simulink model "questao3"  (R2023a)
settings: Solver=VariableStepAuto  StartTime=0.0  StopTime=100  RelTol=1e-3
values from neighbouring files (symbols this model uses):
  B = 0.1    [Trab1_real.m]    (also in questao5.m)
  i0 = 0    [Trab1_real.m]    (also in questao5.m)
  J = 1    [Trab1_real.m]    (also in questao5.m)
  K = 1/3    (= 0.333333333333)    [Trab1_real.m]    (also in questao5.m)
  L = 0.5    [Trab1_real.m]    (also in questao5.m)
  R = 10    [Trab1_real.m]    (also in questao5.m)
settings Model: Creator=pedro  LastModifiedBy=pedro

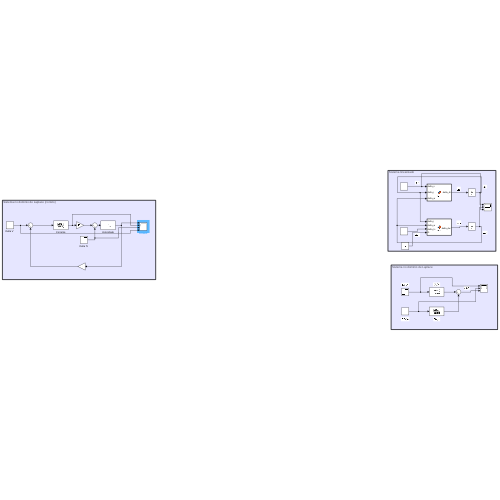
[thumbnail: Simulink's stored preview of the top-level diagram]
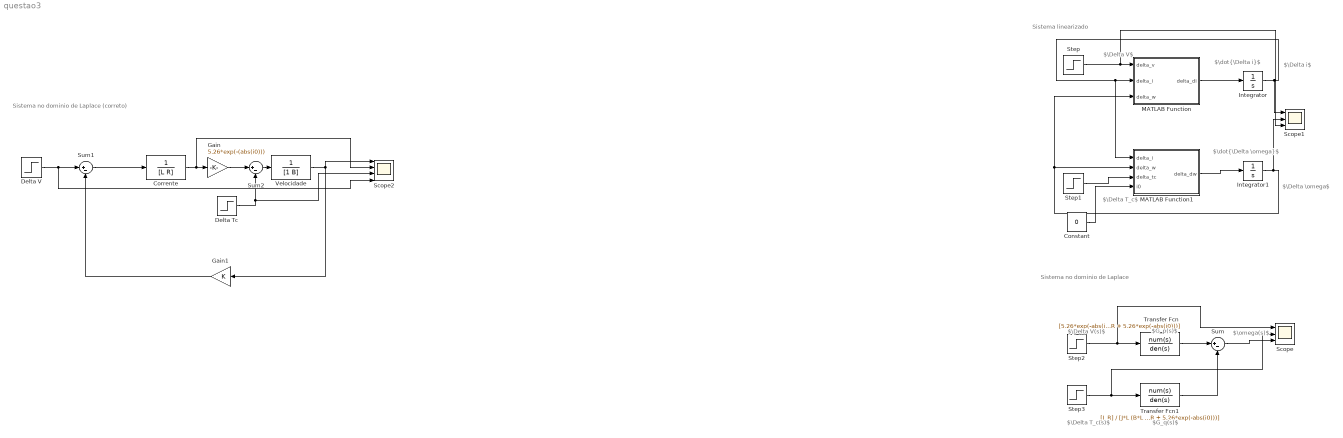
== system questao3 ==
  note: Sistema no dominio de Laplace (correto)
  note: Sistema no dominio de Laplace
  note: $\omega(s)$
  note: $G_q(s)$
  note: $G_p(s)$
  note: $\Delta T_c(s)$
  note: $\Delta V(s)$
  note: $\Delta T_c$
  note: $\Delta V$
  note: $\Delta \omega$
  note: $\dot{\Delta \omega}$
  note: $\Delta i$
  note: $\dot{\Delta i}$
  note: Sistema linearizado
  Constant : Constant  Value=0
  Corrente : TransferFcn  Denominator=[L R]
  Delta Tc : Step  Time=10  After=0.25  SampleTime=0
  "Delta V " : Step  Time=10  After=2  SampleTime=0
  Gain : Gain  Gain=5.26*exp(-(abs(i0)))
  Gain1 : Gain  Gain=K
  Integrator : Integrator
  Integrator1 : Integrator
  MATLAB Function : MATLAB Function  TreatAsAtomicUnit=on
  MATLAB Function1 : MATLAB Function  TreatAsAtomicUnit=on
  Scope : Scope  NumInputPorts=3
  Scope1 : Scope  NumInputPorts=3
  Scope2 : Scope  NumInputPorts=4
  Step : Step  Time=10  After=2  SampleTime=0
  Step1 : Step  Time=10  After=0.25  SampleTime=0
  Step2 : Step  Time=10  After=2  SampleTime=0
  Step3 : Step  Time=10  After=0.25  SampleTime=0
  Sum : Sum  Inputs=|+-
  Sum1 : Sum  Inputs=|+-
  Sum2 : Sum  Inputs=|+-
  Transfer Fcn : TransferFcn  Numerator=[5.26*exp(-abs(i0))]  Denominator=[J*L (B*L + R*J) (B*R + 5.26*exp(-abs(i0)))]
  Transfer Fcn1 : TransferFcn  Numerator=[L R]  Denominator=[J*L (B*L + R*J) (B*R + 5.26*exp(-abs(i0)))]
  Velocidade : TransferFcn  Denominator=[1 B]
  wires:
  MATLAB Function/1(delta_di) -> Integrator/1
  Step/1 -> Scope1/3, MATLAB Function/1(delta_v)
  Integrator/1 -> MATLAB Function1/1(delta_i), MATLAB Function/2(delta_i), Scope1/1
  Step1/1 -> MATLAB Function1/3(delta_tc)
  MATLAB Function1/1(delta_dw) -> Integrator1/1
  Integrator1/1 -> Scope1/2, MATLAB Function1/2(delta_w), MATLAB Function/3(delta_w)
  Step2/1 -> Scope/1, Transfer Fcn/1
  Transfer Fcn/1 -> Sum/1
  Transfer Fcn1/1 -> Sum/2
  Sum/1 -> Scope/3
  Step3/1 -> Scope/2, Transfer Fcn1/1
  Constant/1 -> MATLAB Function1/4(i0)
  "Delta V "/1 -> Scope2/4, Sum1/1
  Sum1/1 -> Corrente/1
  Gain/1 -> Sum2/1
  Delta Tc/1 -> Scope2/3, Sum2/2
  Sum2/1 -> Velocidade/1
  Gain1/1 -> Sum1/2
  Velocidade/1 -> Gain1/1, Scope2/1
  Corrente/1 -> Scope2/2, Gain/1

== matlab function questao3/MATLAB Function1 ==
  data: delta_i input; delta_dw output; delta_w input; delta_tc input; B parameter; J parameter; i0 input
function delta_dw = fcn(delta_i, delta_w, delta_tc, B, J, i0)

delta_dw = (-5.26*exp(-abs(i0))*delta_i - B*delta_w - delta_tc )/(J);

== matlab function questao3/MATLAB Function ==
  data: delta_v input; delta_di output; delta_i input; delta_w input; R parameter; K parameter; L parameter
function delta_di = fcn(delta_v, delta_i, delta_w, R, K, L)

delta_di = (delta_v - R*delta_i - K*delta_w)/(L);
